simulink model "toctest"  (R2016a)
settings: Solver=VariableStepAuto  StartTime=0.0  StopTime=4.0  RelTol=1e-3
undefined symbols (not defined in the file or in its folder): Ts
settings Model: Creator=User  LastModifiedBy=User

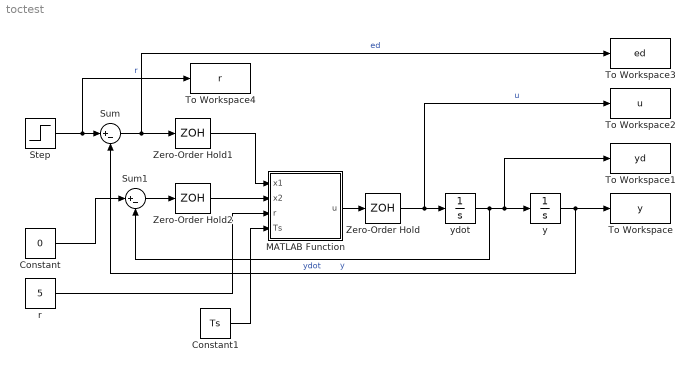
== system toctest ==
  Constant : Constant  Value=0
  Constant1 : Constant  Value=Ts
  MATLAB Function : MATLAB Function  TreatAsAtomicUnit=on
  Step : Step  Time=2  SampleTime=0
  Sum : Sum  Inputs=|+-
  Sum1 : Sum  Inputs=|+-
  To Workspace : ToWorkspace  VariableName=y  SampleTime=-1
  To Workspace1 : ToWorkspace  VariableName=yd  SampleTime=-1
  To Workspace2 : ToWorkspace  VariableName=u  SampleTime=-1
  To Workspace3 : ToWorkspace  VariableName=ed  SampleTime=-1
  To Workspace4 : ToWorkspace  VariableName=r  SampleTime=-1
  Zero-Order Hold : ZeroOrderHold  SampleTime=Ts
  Zero-Order Hold1 : ZeroOrderHold  SampleTime=Ts
  Zero-Order Hold2 : ZeroOrderHold  SampleTime=Ts
  r : Constant  Value=5
  y : Integrator
  ydot : Integrator
  wires:
  Step/1 -> To Workspace4/1, Sum/1  "r"
  r/1 -> MATLAB Function/3(r)
  Constant/1 -> Sum1/1
  ydot/1 -> Sum1/2, To Workspace1/1, y/1  "ydot"
  y/1 -> To Workspace/1, Sum/2  "y"
  MATLAB Function/1(u) -> Zero-Order Hold/1
  Zero-Order Hold/1 -> To Workspace2/1, ydot/1  "u"
  Constant1/1 -> MATLAB Function/4(Ts)
  Sum/1 -> Zero-Order Hold1/1, To Workspace3/1  "ed"
  Sum1/1 -> Zero-Order Hold2/1
  Zero-Order Hold1/1 -> MATLAB Function/1(x1)
  Zero-Order Hold2/1 -> MATLAB Function/2(x2)

== matlab function toctest/MATLAB Function ==
  data: x1 input; x2 input; u output; r input; Ts input
function u = tod(x1,x2,r,Ts)
%#codegen
d = Ts*r;
d0= Ts*d;
y = x1+Ts*x2;
ya=abs(y);
a0= sqrt(d^2 + 8*r*ya);
if (ya > d0),
    a = x2 + (a0-d)/2*sign(y);
else
    a = x2 + y/Ts;
end
aa = abs(a);
if (aa > d),
    fst = r*sign(a);
else
    fst = r*a/d;
end
   
u = fst;
